simulink model "Batterymodel_HiL"  (Simulink 7.8)
settings: Solver=FixedStepDiscrete  SolverMode=SingleTasking  StartTime=0.0  StopTime=inf  FixedStep=T_s  RelTol=1e-3
PreLoadFcn:
  | //BatteryParameters;
  | Init_file_Bat
InitFcn:
  | Init_file_Bat;
values from neighbouring files (symbols this model uses):
  C_diff = 5000    [Init_file_Bat.m]
  CellNo = 12    [Init_file_Bat.m]
  ChargeCurrent = 5    [Init_file_Bat.m]
  ChargeSwitch = 1    [Init_file_Bat.m]
  DischargeCurrent = -5    [Init_file_Bat.m]
  n_cells = 12    [Init_file_Bat.m]
  poles_soc = polyfit(SoC_table, OCV_table,4)    [Init_file_Bat.m]
  Q_0 = 36000*ones(1,12)    [Init_file_Bat.m]
  R_ct = 3.2*10^-3    (= 0.0032)    [Init_file_Bat.m]
  R_diff = 4*10^-3    (= 0.004)    [Init_file_Bat.m]
  R_i = 2*10^-3    (= 0.002)    [Init_file_Bat.m]    (also in Kalman_para_int.m = single(0.05))
  SoCinitCells = SoC_init_cells    [Init_file_Bat.m]
  Tcells = T_cells    [Init_file_Bat.m]
  Ts = 10*10^-3    (= 0.01)    [Init_file_Bat.m]
undefined symbols (not defined in the file or in its folder): DiscIntNeverNeededParam, sigbuilder_block
(part 1 of 2)
settings Model: Creator=wezhang  LastModifiedBy=user  BufferReuse=off
settings OptimizationCC: BlockReduction=off  OptimizeBlockIOStorage=off  BufferReuse=off  ExpressionFolding=off  LocalBlockOutputs=off  InitFltsAndDblsToZero=on  SimCompilerOptimization=On
settings DebuggingCC: FcnCallInpInsideContextMsg=Use local settings
settings HardwareCC: ProdHWDeviceType=Generic->32-bit Embedded Processor
settings SFSimCC: SimParseCustomCode=off
settings RTWCC: SystemTargetFile=lcrt.tlc  GenCodeOnly=on  GenerateMakefile=off  TemplateMakefile=lcrt_default_tmf  GenerateReport=on  ProcessScript=lcrt_make_rtw_hook  LaunchReport=on  RTWCompilerOptimization=On
settings GRTTargetCC: UtilityFuncGeneration=Shared location  MatFileLogging=off  ExtModeMexFile=noextcomm

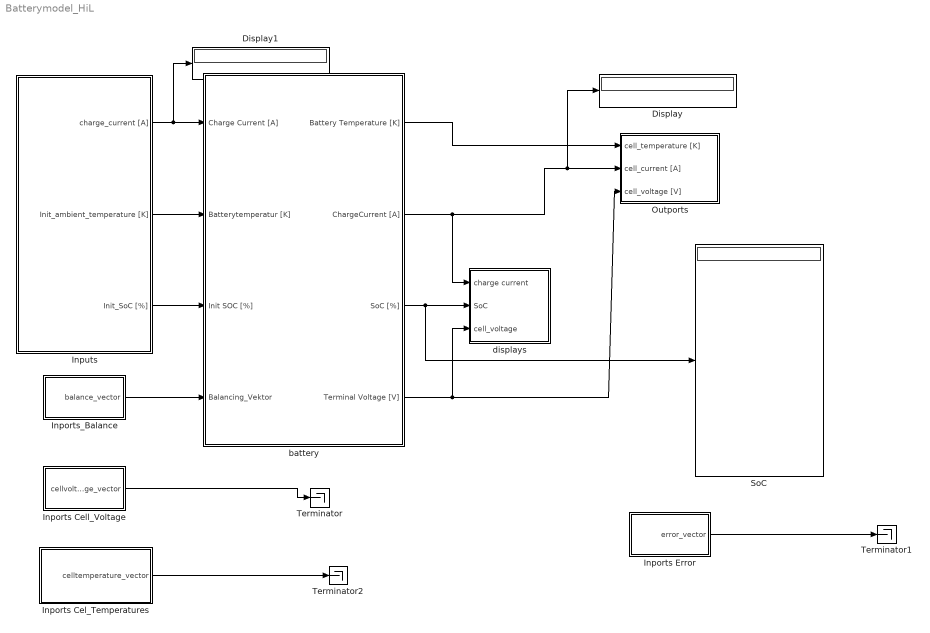
== system Batterymodel_HiL ==
  Display : Display
  Display1 : Display
  Inports Cel_Temperatures : Subsystem
  Inports Cell_Voltage : Subsystem
  Inports Error : Subsystem
  "Inports_Balance " : Subsystem
  Inputs : Subsystem
  Outports : Subsystem
  SoC : Display
  Terminator : Terminator
  Terminator1 : Terminator
  Terminator2 : Terminator
  battery : Subsystem
      settings: MinAlgLoopOccurrences=on
  displays : Subsystem
  wires:
  battery/1(Battery Temperature [K]) -> Outports/1(cell_temperature [K])
  battery/4(Terminal Voltage [V]) -> displays/3(cell_voltage), Outports/3(cell_voltage [V])
  battery/2(ChargeCurrent [A]) -> displays/1(charge current), Outports/2(cell_current [A]), Display/1
  Inputs/1(charge_current [A]) -> battery/1(Charge Current [A]), Display1/1
  Inputs/2(Init_ambient_temperature [K]) -> battery/2(Batterytemperatur [K])
  Inputs/3(Init_SoC [%]) -> battery/3(Init SOC [%])
  battery/3(SoC [%]) -> displays/2(SoC), SoC/1
  Inports Cell_Voltage/1(cellvoltage_vector) -> Terminator/1
  "Inports_Balance "/1(balance_vector) -> battery/4(Balancing_Vektor)
  Inports Error/1(error_vector) -> Terminator1/1
  Inports Cel_Temperatures/1(celltemperature_vector) -> Terminator2/1

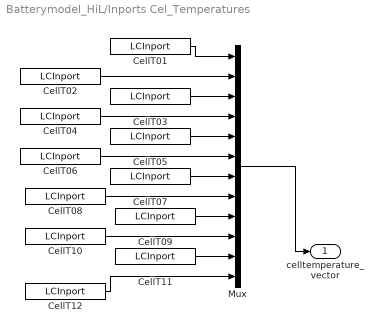
== system Batterymodel_HiL/Inports Cel_Temperatures ==
  CellT01 : S-Function  FunctionName=LCInport  Parameters=ModelName, InportID, b_useConstant, constValue  EnableBusSupport=off  mask(LABCAR Inport){ModelName='Batterymodel_HiL', InportID=0, b_useConstant=0, constValue=0}
      mask prompts: b_useConstant "Use Constant Value if Online"; constValue "Constant Value"
      mask help: This block gets an input to a Simulink model from another module of a LABCAR project
      settings: CopyFcn=set_param( gcb, 'UserData', '####');  OpenFcn=run LCInportGui
      mask Help:
      | Put this block onto any  hierarchy of the model and connect it to the model.
      | Rename it to any suitable name.
      | Then the corresponding signal is available in the Connection Manager for the wiring to any other module..
  CellT02 : S-Function  FunctionName=LCInport  Parameters=ModelName, InportID, b_useConstant, constValue  EnableBusSupport=off  mask(LABCAR Inport){ModelName='Batterymodel_HiL', InportID=1, b_useConstant=0, constValue=0}
      mask prompts: b_useConstant "Use Constant Value if Online"; constValue "Constant Value"
      mask help: This block gets an input to a Simulink model from another module of a LABCAR project
      settings: CopyFcn=set_param( gcb, 'UserData', '####');  OpenFcn=run LCInportGui
      mask Help:
      | Put this block onto any  hierarchy of the model and connect it to the model.
      | Rename it to any suitable name.
      | Then the corresponding signal is available in the Connection Manager for the wiring to any other module..
  CellT03 : S-Function  FunctionName=LCInport  Parameters=ModelName, InportID, b_useConstant, constValue  EnableBusSupport=off  mask(LABCAR Inport){ModelName='Batterymodel_HiL', InportID=2, b_useConstant=0, constValue=0}
      mask prompts: b_useConstant "Use Constant Value if Online"; constValue "Constant Value"
      mask help: This block gets an input to a Simulink model from another module of a LABCAR project
      settings: CopyFcn=set_param( gcb, 'UserData', '####');  OpenFcn=run LCInportGui
      mask Help:
      | Put this block onto any  hierarchy of the model and connect it to the model.
      | Rename it to any suitable name.
      | Then the corresponding signal is available in the Connection Manager for the wiring to any other module..
  CellT04 : S-Function  FunctionName=LCInport  Parameters=ModelName, InportID, b_useConstant, constValue  EnableBusSupport=off  mask(LABCAR Inport){ModelName='Batterymodel_HiL', InportID=3, b_useConstant=0, constValue=0}
      mask prompts: b_useConstant "Use Constant Value if Online"; constValue "Constant Value"
      mask help: This block gets an input to a Simulink model from another module of a LABCAR project
      settings: CopyFcn=set_param( gcb, 'UserData', '####');  OpenFcn=run LCInportGui
      mask Help:
      | Put this block onto any  hierarchy of the model and connect it to the model.
      | Rename it to any suitable name.
      | Then the corresponding signal is available in the Connection Manager for the wiring to any other module..
  CellT05 : S-Function  FunctionName=LCInport  Parameters=ModelName, InportID, b_useConstant, constValue  EnableBusSupport=off  mask(LABCAR Inport){ModelName='Batterymodel_HiL', InportID=4, b_useConstant=0, constValue=0}
      mask prompts: b_useConstant "Use Constant Value if Online"; constValue "Constant Value"
      mask help: This block gets an input to a Simulink model from another module of a LABCAR project
      settings: CopyFcn=set_param( gcb, 'UserData', '####');  OpenFcn=run LCInportGui
      mask Help:
      | Put this block onto any  hierarchy of the model and connect it to the model.
      | Rename it to any suitable name.
      | Then the corresponding signal is available in the Connection Manager for the wiring to any other module..
  CellT06 : S-Function  FunctionName=LCInport  Parameters=ModelName, InportID, b_useConstant, constValue  EnableBusSupport=off  mask(LABCAR Inport){ModelName='Batterymodel_HiL', InportID=5, b_useConstant=0, constValue=0}
      mask prompts: b_useConstant "Use Constant Value if Online"; constValue "Constant Value"
      mask help: This block gets an input to a Simulink model from another module of a LABCAR project
      settings: CopyFcn=set_param( gcb, 'UserData', '####');  OpenFcn=run LCInportGui
      mask Help:
      | Put this block onto any  hierarchy of the model and connect it to the model.
      | Rename it to any suitable name.
      | Then the corresponding signal is available in the Connection Manager for the wiring to any other module..
  CellT07 : S-Function  FunctionName=LCInport  Parameters=ModelName, InportID, b_useConstant, constValue  EnableBusSupport=off  mask(LABCAR Inport){ModelName='Batterymodel_HiL', InportID=6, b_useConstant=0, constValue=0}
      mask prompts: b_useConstant "Use Constant Value if Online"; constValue "Constant Value"
      mask help: This block gets an input to a Simulink model from another module of a LABCAR project
      settings: CopyFcn=set_param( gcb, 'UserData', '####');  OpenFcn=run LCInportGui
      mask Help:
      | Put this block onto any  hierarchy of the model and connect it to the model.
      | Rename it to any suitable name.
      | Then the corresponding signal is available in the Connection Manager for the wiring to any other module..
  CellT08 : S-Function  FunctionName=LCInport  Parameters=ModelName, InportID, b_useConstant, constValue  EnableBusSupport=off  mask(LABCAR Inport){ModelName='Batterymodel_HiL', InportID=7, b_useConstant=0, constValue=0}
      mask prompts: b_useConstant "Use Constant Value if Online"; constValue "Constant Value"
      mask help: This block gets an input to a Simulink model from another module of a LABCAR project
      settings: CopyFcn=set_param( gcb, 'UserData', '####');  OpenFcn=run LCInportGui
      mask Help:
      | Put this block onto any  hierarchy of the model and connect it to the model.
      | Rename it to any suitable name.
      | Then the corresponding signal is available in the Connection Manager for the wiring to any other module..
  CellT09 : S-Function  FunctionName=LCInport  Parameters=ModelName, InportID, b_useConstant, constValue  EnableBusSupport=off  mask(LABCAR Inport){ModelName='Batterymodel_HiL', InportID=8, b_useConstant=0, constValue=0}
      mask prompts: b_useConstant "Use Constant Value if Online"; constValue "Constant Value"
      mask help: This block gets an input to a Simulink model from another module of a LABCAR project
      settings: CopyFcn=set_param( gcb, 'UserData', '####');  OpenFcn=run LCInportGui
      mask Help:
      | Put this block onto any  hierarchy of the model and connect it to the model.
      | Rename it to any suitable name.
      | Then the corresponding signal is available in the Connection Manager for the wiring to any other module..
  CellT10 : S-Function  FunctionName=LCInport  Parameters=ModelName, InportID, b_useConstant, constValue  EnableBusSupport=off  mask(LABCAR Inport){ModelName='Batterymodel_HiL', InportID=9, b_useConstant=0, constValue=0}
      mask prompts: b_useConstant "Use Constant Value if Online"; constValue "Constant Value"
      mask help: This block gets an input to a Simulink model from another module of a LABCAR project
      settings: CopyFcn=set_param( gcb, 'UserData', '####');  OpenFcn=run LCInportGui
      mask Help:
      | Put this block onto any  hierarchy of the model and connect it to the model.
      | Rename it to any suitable name.
      | Then the corresponding signal is available in the Connection Manager for the wiring to any other module..
  CellT11 : S-Function  FunctionName=LCInport  Parameters=ModelName, InportID, b_useConstant, constValue  EnableBusSupport=off  mask(LABCAR Inport){ModelName='Batterymodel_HiL', InportID=10, b_useConstant=0, constValue=0}
      mask prompts: b_useConstant "Use Constant Value if Online"; constValue "Constant Value"
      mask help: This block gets an input to a Simulink model from another module of a LABCAR project
      settings: CopyFcn=set_param( gcb, 'UserData', '####');  OpenFcn=run LCInportGui
      mask Help:
      | Put this block onto any  hierarchy of the model and connect it to the model.
      | Rename it to any suitable name.
      | Then the corresponding signal is available in the Connection Manager for the wiring to any other module..
  CellT12 : S-Function  FunctionName=LCInport  Parameters=ModelName, InportID, b_useConstant, constValue  EnableBusSupport=off  mask(LABCAR Inport){ModelName='Batterymodel_HiL', InportID=11, b_useConstant=0, constValue=0}
      mask prompts: b_useConstant "Use Constant Value if Online"; constValue "Constant Value"
      mask help: This block gets an input to a Simulink model from another module of a LABCAR project
      settings: CopyFcn=set_param( gcb, 'UserData', '####');  OpenFcn=run LCInportGui
      mask Help:
      | Put this block onto any  hierarchy of the model and connect it to the model.
      | Rename it to any suitable name.
      | Then the corresponding signal is available in the Connection Manager for the wiring to any other module..
  Mux : Mux  Inputs=12
  celltemperature_vector : Outport
  wires:
  CellT01/1 -> Mux/1
  CellT02/1 -> Mux/2
  CellT03/1 -> Mux/3
  CellT04/1 -> Mux/4
  CellT05/1 -> Mux/5
  CellT06/1 -> Mux/6
  CellT08/1 -> Mux/8
  CellT10/1 -> Mux/10
  CellT12/1 -> Mux/12
  CellT11/1 -> Mux/11
  CellT09/1 -> Mux/9
  CellT07/1 -> Mux/7
  Mux/1 -> celltemperature_vector/1

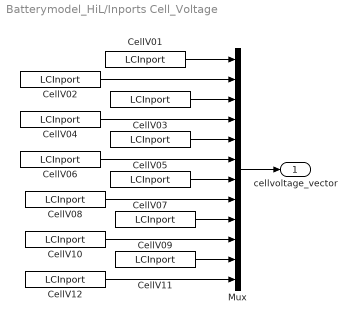
== system Batterymodel_HiL/Inports Cell_Voltage ==
  CellV01 : S-Function  FunctionName=LCInport  Parameters=ModelName, InportID, b_useConstant, constValue  EnableBusSupport=off  mask(LABCAR Inport){ModelName='Batterymodel_HiL', InportID=12, b_useConstant=0, constValue=0}
      mask prompts: b_useConstant "Use Constant Value if Online"; constValue "Constant Value"
      mask help: This block gets an input to a Simulink model from another module of a LABCAR project
      settings: CopyFcn=set_param( gcb, 'UserData', '####');  OpenFcn=run LCInportGui
      mask Help:
      | Put this block onto any  hierarchy of the model and connect it to the model.
      | Rename it to any suitable name.
      | Then the corresponding signal is available in the Connection Manager for the wiring to any other module..
  CellV02 : S-Function  FunctionName=LCInport  Parameters=ModelName, InportID, b_useConstant, constValue  EnableBusSupport=off  mask(LABCAR Inport){ModelName='Batterymodel_HiL', InportID=13, b_useConstant=0, constValue=0}
      mask prompts: b_useConstant "Use Constant Value if Online"; constValue "Constant Value"
      mask help: This block gets an input to a Simulink model from another module of a LABCAR project
      settings: CopyFcn=set_param( gcb, 'UserData', '####');  OpenFcn=run LCInportGui
      mask Help:
      | Put this block onto any  hierarchy of the model and connect it to the model.
      | Rename it to any suitable name.
      | Then the corresponding signal is available in the Connection Manager for the wiring to any other module..
  CellV03 : S-Function  FunctionName=LCInport  Parameters=ModelName, InportID, b_useConstant, constValue  EnableBusSupport=off  mask(LABCAR Inport){ModelName='Batterymodel_HiL', InportID=14, b_useConstant=0, constValue=0}
      mask prompts: b_useConstant "Use Constant Value if Online"; constValue "Constant Value"
      mask help: This block gets an input to a Simulink model from another module of a LABCAR project
      settings: CopyFcn=set_param( gcb, 'UserData', '####');  OpenFcn=run LCInportGui
      mask Help:
      | Put this block onto any  hierarchy of the model and connect it to the model.
      | Rename it to any suitable name.
      | Then the corresponding signal is available in the Connection Manager for the wiring to any other module..
  CellV04 : S-Function  FunctionName=LCInport  Parameters=ModelName, InportID, b_useConstant, constValue  EnableBusSupport=off  mask(LABCAR Inport){ModelName='Batterymodel_HiL', InportID=15, b_useConstant=0, constValue=0}
      mask prompts: b_useConstant "Use Constant Value if Online"; constValue "Constant Value"
      mask help: This block gets an input to a Simulink model from another module of a LABCAR project
      settings: CopyFcn=set_param( gcb, 'UserData', '####');  OpenFcn=run LCInportGui
      mask Help:
      | Put this block onto any  hierarchy of the model and connect it to the model.
      | Rename it to any suitable name.
      | Then the corresponding signal is available in the Connection Manager for the wiring to any other module..
  CellV05 : S-Function  FunctionName=LCInport  Parameters=ModelName, InportID, b_useConstant, constValue  EnableBusSupport=off  mask(LABCAR Inport){ModelName='Batterymodel_HiL', InportID=16, b_useConstant=0, constValue=0}
      mask prompts: b_useConstant "Use Constant Value if Online"; constValue "Constant Value"
      mask help: This block gets an input to a Simulink model from another module of a LABCAR project
      settings: CopyFcn=set_param( gcb, 'UserData', '####');  OpenFcn=run LCInportGui
      mask Help:
      | Put this block onto any  hierarchy of the model and connect it to the model.
      | Rename it to any suitable name.
      | Then the corresponding signal is available in the Connection Manager for the wiring to any other module..
  CellV06 : S-Function  FunctionName=LCInport  Parameters=ModelName, InportID, b_useConstant, constValue  EnableBusSupport=off  mask(LABCAR Inport){ModelName='Batterymodel_HiL', InportID=17, b_useConstant=0, constValue=0}
      mask prompts: b_useConstant "Use Constant Value if Online"; constValue "Constant Value"
      mask help: This block gets an input to a Simulink model from another module of a LABCAR project
      settings: CopyFcn=set_param( gcb, 'UserData', '####');  OpenFcn=run LCInportGui
      mask Help:
      | Put this block onto any  hierarchy of the model and connect it to the model.
      | Rename it to any suitable name.
      | Then the corresponding signal is available in the Connection Manager for the wiring to any other module..
  CellV07 : S-Function  FunctionName=LCInport  Parameters=ModelName, InportID, b_useConstant, constValue  EnableBusSupport=off  mask(LABCAR Inport){ModelName='Batterymodel_HiL', InportID=18, b_useConstant=0, constValue=0}
      mask prompts: b_useConstant "Use Constant Value if Online"; constValue "Constant Value"
      mask help: This block gets an input to a Simulink model from another module of a LABCAR project
      settings: CopyFcn=set_param( gcb, 'UserData', '####');  OpenFcn=run LCInportGui
      mask Help:
      | Put this block onto any  hierarchy of the model and connect it to the model.
      | Rename it to any suitable name.
      | Then the corresponding signal is available in the Connection Manager for the wiring to any other module..
  CellV08 : S-Function  FunctionName=LCInport  Parameters=ModelName, InportID, b_useConstant, constValue  EnableBusSupport=off  mask(LABCAR Inport){ModelName='Batterymodel_HiL', InportID=19, b_useConstant=0, constValue=0}
      mask prompts: b_useConstant "Use Constant Value if Online"; constValue "Constant Value"
      mask help: This block gets an input to a Simulink model from another module of a LABCAR project
      settings: CopyFcn=set_param( gcb, 'UserData', '####');  OpenFcn=run LCInportGui
      mask Help:
      | Put this block onto any  hierarchy of the model and connect it to the model.
      | Rename it to any suitable name.
      | Then the corresponding signal is available in the Connection Manager for the wiring to any other module..
  CellV09 : S-Function  FunctionName=LCInport  Parameters=ModelName, InportID, b_useConstant, constValue  EnableBusSupport=off  mask(LABCAR Inport){ModelName='Batterymodel_HiL', InportID=20, b_useConstant=0, constValue=0}
      mask prompts: b_useConstant "Use Constant Value if Online"; constValue "Constant Value"
      mask help: This block gets an input to a Simulink model from another module of a LABCAR project
      settings: CopyFcn=set_param( gcb, 'UserData', '####');  OpenFcn=run LCInportGui
      mask Help:
      | Put this block onto any  hierarchy of the model and connect it to the model.
      | Rename it to any suitable name.
      | Then the corresponding signal is available in the Connection Manager for the wiring to any other module..
  CellV10 : S-Function  FunctionName=LCInport  Parameters=ModelName, InportID, b_useConstant, constValue  EnableBusSupport=off  mask(LABCAR Inport){ModelName='Batterymodel_HiL', InportID=21, b_useConstant=0, constValue=0}
      mask prompts: b_useConstant "Use Constant Value if Online"; constValue "Constant Value"
      mask help: This block gets an input to a Simulink model from another module of a LABCAR project
      settings: CopyFcn=set_param( gcb, 'UserData', '####');  OpenFcn=run LCInportGui
      mask Help:
      | Put this block onto any  hierarchy of the model and connect it to the model.
      | Rename it to any suitable name.
      | Then the corresponding signal is available in the Connection Manager for the wiring to any other module..
  CellV11 : S-Function  FunctionName=LCInport  Parameters=ModelName, InportID, b_useConstant, constValue  EnableBusSupport=off  mask(LABCAR Inport){ModelName='Batterymodel_HiL', InportID=22, b_useConstant=0, constValue=0}
      mask prompts: b_useConstant "Use Constant Value if Online"; constValue "Constant Value"
      mask help: This block gets an input to a Simulink model from another module of a LABCAR project
      settings: CopyFcn=set_param( gcb, 'UserData', '####');  OpenFcn=run LCInportGui
      mask Help:
      | Put this block onto any  hierarchy of the model and connect it to the model.
      | Rename it to any suitable name.
      | Then the corresponding signal is available in the Connection Manager for the wiring to any other module..
  CellV12 : S-Function  FunctionName=LCInport  Parameters=ModelName, InportID, b_useConstant, constValue  EnableBusSupport=off  mask(LABCAR Inport){ModelName='Batterymodel_HiL', InportID=23, b_useConstant=0, constValue=0}
      mask prompts: b_useConstant "Use Constant Value if Online"; constValue "Constant Value"
      mask help: This block gets an input to a Simulink model from another module of a LABCAR project
      settings: CopyFcn=set_param( gcb, 'UserData', '####');  OpenFcn=run LCInportGui
      mask Help:
      | Put this block onto any  hierarchy of the model and connect it to the model.
      | Rename it to any suitable name.
      | Then the corresponding signal is available in the Connection Manager for the wiring to any other module..
  Mux : Mux  Inputs=12
  cellvoltage_vector : Outport
  wires:
  CellV01/1 -> Mux/1
  CellV02/1 -> Mux/2
  CellV03/1 -> Mux/3
  CellV04/1 -> Mux/4
  CellV05/1 -> Mux/5
  CellV06/1 -> Mux/6
  CellV08/1 -> Mux/8
  CellV10/1 -> Mux/10
  CellV12/1 -> Mux/12
  CellV11/1 -> Mux/11
  CellV09/1 -> Mux/9
  CellV07/1 -> Mux/7
  Mux/1 -> cellvoltage_vector/1

== system Batterymodel_HiL/Inports Error ==
  Error_CellNo : S-Function  FunctionName=LCInport  Parameters=ModelName, InportID, b_useConstant, constValue  EnableBusSupport=off  mask(LABCAR Inport){ModelName='Batterymodel_HiL', InportID=24, b_useConstant=0, constValue=0}
      mask prompts: b_useConstant "Use Constant Value if Online"; constValue "Constant Value"
      mask help: This block gets an input to a Simulink model from another module of a LABCAR project
      settings: CopyFcn=set_param( gcb, 'UserData', '####');  OpenFcn=run LCInportGui
      mask Help:
      | Put this block onto any  hierarchy of the model and connect it to the model.
      | Rename it to any suitable name.
      | Then the corresponding signal is available in the Connection Manager for the wiring to any other module..
  Error_Event : S-Function  FunctionName=LCInport  Parameters=ModelName, InportID, b_useConstant, constValue  EnableBusSupport=off  mask(LABCAR Inport){ModelName='Batterymodel_HiL', InportID=25, b_useConstant=0, constValue=0}
      mask prompts: b_useConstant "Use Constant Value if Online"; constValue "Constant Value"
      mask help: This block gets an input to a Simulink model from another module of a LABCAR project
      settings: CopyFcn=set_param( gcb, 'UserData', '####');  OpenFcn=run LCInportGui
      mask Help:
      | Put this block onto any  hierarchy of the model and connect it to the model.
      | Rename it to any suitable name.
      | Then the corresponding signal is available in the Connection Manager for the wiring to any other module..
  Error_Indication : S-Function  FunctionName=LCInport  Parameters=ModelName, InportID, b_useConstant, constValue  EnableBusSupport=off  mask(LABCAR Inport){ModelName='Batterymodel_HiL', InportID=26, b_useConstant=0, constValue=0}
      mask prompts: b_useConstant "Use Constant Value if Online"; constValue "Constant Value"
      mask help: This block gets an input to a Simulink model from another module of a LABCAR project
      settings: CopyFcn=set_param( gcb, 'UserData', '####');  OpenFcn=run LCInportGui
      mask Help:
      | Put this block onto any  hierarchy of the model and connect it to the model.
      | Rename it to any suitable name.
      | Then the corresponding signal is available in the Connection Manager for the wiring to any other module..
  Mux : Mux  Inputs=3
  error_vector : Outport
  wires:
  Error_Indication/1 -> Mux/1
  Error_Event/1 -> Mux/2
  Error_CellNo/1 -> Mux/3
  Mux/1 -> error_vector/1

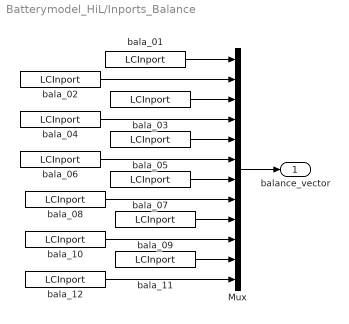
== system Batterymodel_HiL/Inports_Balance  ==
  Mux : Mux  Inputs=12
  bala_01 : S-Function  FunctionName=LCInport  Parameters=ModelName, InportID, b_useConstant, constValue  EnableBusSupport=off  mask(LABCAR Inport){ModelName='Batterymodel_HiL', InportID=27, b_useConstant=0, constValue=0}
      mask prompts: b_useConstant "Use Constant Value if Online"; constValue "Constant Value"
      mask help: This block gets an input to a Simulink model from another module of a LABCAR project
      settings: CopyFcn=set_param( gcb, 'UserData', '####');  OpenFcn=run LCInportGui
      mask Help:
      | Put this block onto any  hierarchy of the model and connect it to the model.
      | Rename it to any suitable name.
      | Then the corresponding signal is available in the Connection Manager for the wiring to any other module..
  bala_02 : S-Function  FunctionName=LCInport  Parameters=ModelName, InportID, b_useConstant, constValue  EnableBusSupport=off  mask(LABCAR Inport){ModelName='Batterymodel_HiL', InportID=28, b_useConstant=0, constValue=0}
      mask prompts: b_useConstant "Use Constant Value if Online"; constValue "Constant Value"
      mask help: This block gets an input to a Simulink model from another module of a LABCAR project
      settings: CopyFcn=set_param( gcb, 'UserData', '####');  OpenFcn=run LCInportGui
      mask Help:
      | Put this block onto any  hierarchy of the model and connect it to the model.
      | Rename it to any suitable name.
      | Then the corresponding signal is available in the Connection Manager for the wiring to any other module..
  bala_03 : S-Function  FunctionName=LCInport  Parameters=ModelName, InportID, b_useConstant, constValue  EnableBusSupport=off  mask(LABCAR Inport){ModelName='Batterymodel_HiL', InportID=29, b_useConstant=0, constValue=0}
      mask prompts: b_useConstant "Use Constant Value if Online"; constValue "Constant Value"
      mask help: This block gets an input to a Simulink model from another module of a LABCAR project
      settings: CopyFcn=set_param( gcb, 'UserData', '####');  OpenFcn=run LCInportGui
      mask Help:
      | Put this block onto any  hierarchy of the model and connect it to the model.
      | Rename it to any suitable name.
      | Then the corresponding signal is available in the Connection Manager for the wiring to any other module..
  bala_04 : S-Function  FunctionName=LCInport  Parameters=ModelName, InportID, b_useConstant, constValue  EnableBusSupport=off  mask(LABCAR Inport){ModelName='Batterymodel_HiL', InportID=30, b_useConstant=0, constValue=0}
      mask prompts: b_useConstant "Use Constant Value if Online"; constValue "Constant Value"
      mask help: This block gets an input to a Simulink model from another module of a LABCAR project
      settings: CopyFcn=set_param( gcb, 'UserData', '####');  OpenFcn=run LCInportGui
      mask Help:
      | Put this block onto any  hierarchy of the model and connect it to the model.
      | Rename it to any suitable name.
      | Then the corresponding signal is available in the Connection Manager for the wiring to any other module..
  bala_05 : S-Function  FunctionName=LCInport  Parameters=ModelName, InportID, b_useConstant, constValue  EnableBusSupport=off  mask(LABCAR Inport){ModelName='Batterymodel_HiL', InportID=31, b_useConstant=0, constValue=0}
      mask prompts: b_useConstant "Use Constant Value if Online"; constValue "Constant Value"
      mask help: This block gets an input to a Simulink model from another module of a LABCAR project
      settings: CopyFcn=set_param( gcb, 'UserData', '####');  OpenFcn=run LCInportGui
      mask Help:
      | Put this block onto any  hierarchy of the model and connect it to the model.
      | Rename it to any suitable name.
      | Then the corresponding signal is available in the Connection Manager for the wiring to any other module..
  bala_06 : S-Function  FunctionName=LCInport  Parameters=ModelName, InportID, b_useConstant, constValue  EnableBusSupport=off  mask(LABCAR Inport){ModelName='Batterymodel_HiL', InportID=32, b_useConstant=0, constValue=0}
      mask prompts: b_useConstant "Use Constant Value if Online"; constValue "Constant Value"
      mask help: This block gets an input to a Simulink model from another module of a LABCAR project
      settings: CopyFcn=set_param( gcb, 'UserData', '####');  OpenFcn=run LCInportGui
      mask Help:
      | Put this block onto any  hierarchy of the model and connect it to the model.
      | Rename it to any suitable name.
      | Then the corresponding signal is available in the Connection Manager for the wiring to any other module..
  bala_07 : S-Function  FunctionName=LCInport  Parameters=ModelName, InportID, b_useConstant, constValue  EnableBusSupport=off  mask(LABCAR Inport){ModelName='Batterymodel_HiL', InportID=33, b_useConstant=0, constValue=0}
      mask prompts: b_useConstant "Use Constant Value if Online"; constValue "Constant Value"
      mask help: This block gets an input to a Simulink model from another module of a LABCAR project
      settings: CopyFcn=set_param( gcb, 'UserData', '####');  OpenFcn=run LCInportGui
      mask Help:
      | Put this block onto any  hierarchy of the model and connect it to the model.
      | Rename it to any suitable name.
      | Then the corresponding signal is available in the Connection Manager for the wiring to any other module..
  bala_08 : S-Function  FunctionName=LCInport  Parameters=ModelName, InportID, b_useConstant, constValue  EnableBusSupport=off  mask(LABCAR Inport){ModelName='Batterymodel_HiL', InportID=34, b_useConstant=0, constValue=0}
      mask prompts: b_useConstant "Use Constant Value if Online"; constValue "Constant Value"
      mask help: This block gets an input to a Simulink model from another module of a LABCAR project
      settings: CopyFcn=set_param( gcb, 'UserData', '####');  OpenFcn=run LCInportGui
      mask Help:
      | Put this block onto any  hierarchy of the model and connect it to the model.
      | Rename it to any suitable name.
      | Then the corresponding signal is available in the Connection Manager for the wiring to any other module..
  bala_09 : S-Function  FunctionName=LCInport  Parameters=ModelName, InportID, b_useConstant, constValue  EnableBusSupport=off  mask(LABCAR Inport){ModelName='Batterymodel_HiL', InportID=35, b_useConstant=0, constValue=0}
      mask prompts: b_useConstant "Use Constant Value if Online"; constValue "Constant Value"
      mask help: This block gets an input to a Simulink model from another module of a LABCAR project
      settings: CopyFcn=set_param( gcb, 'UserData', '####');  OpenFcn=run LCInportGui
      mask Help:
      | Put this block onto any  hierarchy of the model and connect it to the model.
      | Rename it to any suitable name.
      | Then the corresponding signal is available in the Connection Manager for the wiring to any other module..
  bala_10 : S-Function  FunctionName=LCInport  Parameters=ModelName, InportID, b_useConstant, constValue  EnableBusSupport=off  mask(LABCAR Inport){ModelName='Batterymodel_HiL', InportID=36, b_useConstant=0, constValue=0}
      mask prompts: b_useConstant "Use Constant Value if Online"; constValue "Constant Value"
      mask help: This block gets an input to a Simulink model from another module of a LABCAR project
      settings: CopyFcn=set_param( gcb, 'UserData', '####');  OpenFcn=run LCInportGui
      mask Help:
      | Put this block onto any  hierarchy of the model and connect it to the model.
      | Rename it to any suitable name.
      | Then the corresponding signal is available in the Connection Manager for the wiring to any other module..
  bala_11 : S-Function  FunctionName=LCInport  Parameters=ModelName, InportID, b_useConstant, constValue  EnableBusSupport=off  mask(LABCAR Inport){ModelName='Batterymodel_HiL', InportID=37, b_useConstant=0, constValue=0}
      mask prompts: b_useConstant "Use Constant Value if Online"; constValue "Constant Value"
      mask help: This block gets an input to a Simulink model from another module of a LABCAR project
      settings: CopyFcn=set_param( gcb, 'UserData', '####');  OpenFcn=run LCInportGui
      mask Help:
      | Put this block onto any  hierarchy of the model and connect it to the model.
      | Rename it to any suitable name.
      | Then the corresponding signal is available in the Connection Manager for the wiring to any other module..
  bala_12 : S-Function  FunctionName=LCInport  Parameters=ModelName, InportID, b_useConstant, constValue  EnableBusSupport=off  mask(LABCAR Inport){ModelName='Batterymodel_HiL', InportID=38, b_useConstant=0, constValue=0}
      mask prompts: b_useConstant "Use Constant Value if Online"; constValue "Constant Value"
      mask help: This block gets an input to a Simulink model from another module of a LABCAR project
      settings: CopyFcn=set_param( gcb, 'UserData', '####');  OpenFcn=run LCInportGui
      mask Help:
      | Put this block onto any  hierarchy of the model and connect it to the model.
      | Rename it to any suitable name.
      | Then the corresponding signal is available in the Connection Manager for the wiring to any other module..
  balance_vector : Outport
  wires:
  bala_01/1 -> Mux/1
  bala_02/1 -> Mux/2
  bala_03/1 -> Mux/3
  bala_04/1 -> Mux/4
  bala_05/1 -> Mux/5
  bala_06/1 -> Mux/6
  bala_08/1 -> Mux/8
  bala_10/1 -> Mux/10
  bala_12/1 -> Mux/12
  bala_11/1 -> Mux/11
  bala_09/1 -> Mux/9
  bala_07/1 -> Mux/7
  Mux/1 -> balance_vector/1

== system Batterymodel_HiL/Inputs ==
  Betriebsmodus : Subsystem
  Charge Profile : Subsystem
  Init Ambient Temperature [K] : Constant  Value=Tcells
  Init SoC [%] : Constant  Value=SoCinitCells
  charge_current [A] : Outport
  Init_ambient_temperature [K] : Outport  Port=2
  Init_SoC [%] : Outport  Port=3
  wires:
  Charge Profile/1(Current [A]) -> charge_current [A]/1
  Init Ambient Temperature [K]/1 -> Init_ambient_temperature [K]/1
  Init SoC [%]/1 -> Init_SoC [%]/1

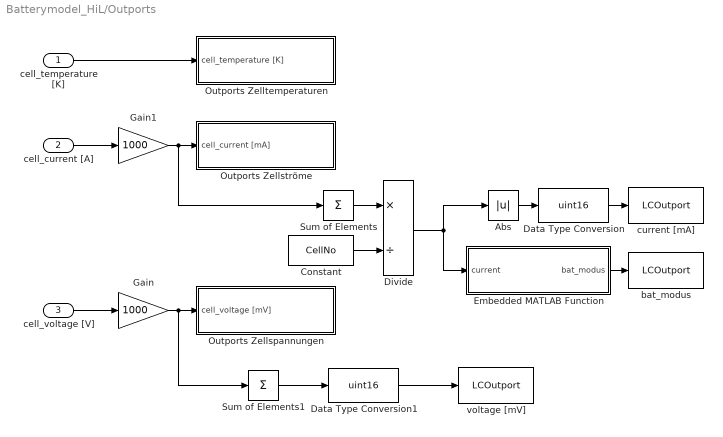
== system Batterymodel_HiL/Outports ==
  cell_temperature [K] : Inport
  cell_current [A] : Inport  Port=2
  cell_voltage [V] : Inport  Port=3
  Abs : Abs
  Constant : Constant  Value=CellNo
  Data Type Conversion : DataTypeConversion  OutDataTypeStr=uint16
  Data Type Conversion1 : DataTypeConversion  OutDataTypeStr=uint16
  Divide : Product  Inputs=*/
  Embedded MATLAB Function : MATLAB Function  TreatAsAtomicUnit=on
  Gain : Gain  Gain=1000
  Gain1 : Gain  Gain=1000
  Outports Zellspannungen : Subsystem
  Outports Zellströme : Subsystem
  Outports Zelltemperaturen : Subsystem
  Sum of Elements : Sum  Inputs=+
  Sum of Elements1 : Sum  Inputs=+
  bat_modus : S-Function  FunctionName=LCOutport  Parameters=ModelName, OutportID  EnableBusSupport=off  mask(LABCAR Outport){ModelName='Batterymodel_HiL', OutportID=37}
      mask help: This block defines an output of a Simulink model to another module of a LABCAR project
      settings: CopyFcn=set_param( gcb, 'UserData', '####');  OpenFcn=LCOpenFcnCallback
      mask Help:
      | Put this block onto any  hierarchy of the model and connect it to the model.
      | Rename it to any suitable name.
      | Then the corresponding signal is available in the Connection Manager for the wiring to any other module..
  current [mA] : S-Function  FunctionName=LCOutport  Parameters=ModelName, OutportID  EnableBusSupport=off  mask(LABCAR Outport){ModelName='Batterymodel_HiL', OutportID=38}
      mask help: This block defines an output of a Simulink model to another module of a LABCAR project
      settings: CopyFcn=set_param( gcb, 'UserData', '####');  OpenFcn=LCOpenFcnCallback
      mask Help:
      | Put this block onto any  hierarchy of the model and connect it to the model.
      | Rename it to any suitable name.
      | Then the corresponding signal is available in the Connection Manager for the wiring to any other module..
  voltage [mV] : S-Function  FunctionName=LCOutport  Parameters=ModelName, OutportID  EnableBusSupport=off  mask(LABCAR Outport){ModelName='Batterymodel_HiL', OutportID=39}
      mask help: This block defines an output of a Simulink model to another module of a LABCAR project
      settings: CopyFcn=set_param( gcb, 'UserData', '####');  OpenFcn=LCOpenFcnCallback
      mask Help:
      | Put this block onto any  hierarchy of the model and connect it to the model.
      | Rename it to any suitable name.
      | Then the corresponding signal is available in the Connection Manager for the wiring to any other module..
  wires:
  Gain/1 -> Outports Zellspannungen/1(cell_voltage [mV]), Sum of Elements1/1
  cell_voltage [V]/1 -> Gain/1
  cell_temperature [K]/1 -> Outports Zelltemperaturen/1(cell_temperature [K])
  cell_current [A]/1 -> Gain1/1
  Sum of Elements/1 -> Divide/1
  Constant/1 -> Divide/2
  Gain1/1 -> Outports Zellströme/1(cell_current [mA]), Sum of Elements/1
  Sum of Elements1/1 -> Data Type Conversion1/1
  Abs/1 -> Data Type Conversion/1
  Divide/1 -> Embedded MATLAB Function/1(current), Abs/1
  Embedded MATLAB Function/1(bat_modus) -> bat_modus/1
  Data Type Conversion/1 -> current [mA]/1
  Data Type Conversion1/1 -> voltage [mV]/1

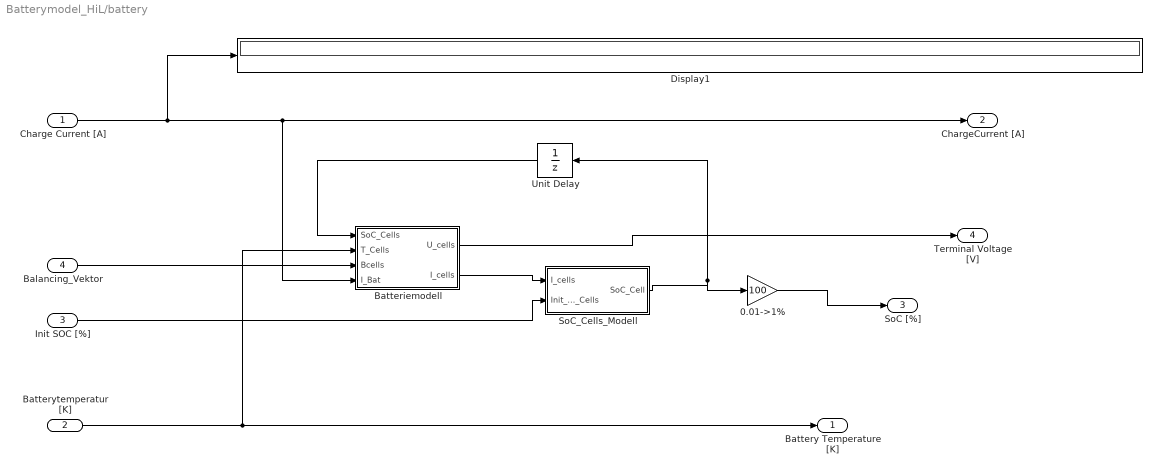
== system Batterymodel_HiL/battery ==
  Charge Current [A] : Inport
  Batterytemperatur [K] : Inport  Port=2
  Init SOC [%] : Inport  Port=3
  Balancing_Vektor : Inport  Port=4
  0.01->1% : Gain  Gain=100
  Batteriemodell : Subsystem
  Display1 : Display
  SoC_Cells_Modell : Subsystem
  Unit Delay : UnitDelay  SampleTime=-1
  Battery Temperature [K] : Outport
  ChargeCurrent [A] : Outport  Port=2
  SoC [%] : Outport  Port=3
  Terminal Voltage [V] : Outport  Port=4
  wires:
  Charge Current [A]/1 -> Batteriemodell/4(I_Bat), ChargeCurrent [A]/1, Display1/1
  Batteriemodell/2(I_cells) -> SoC_Cells_Modell/1(I_cells)
  SoC_Cells_Modell/1(SoC_Cell) -> Unit Delay/1, 0.01->1%/1
  Batteriemodell/1(U_cells) -> Terminal Voltage [V]/1
  Batterytemperatur [K]/1 -> Batteriemodell/2(T_Cells), Battery Temperature [K]/1
  Init SOC [%]/1 -> SoC_Cells_Modell/2(Init_SoC_Cells)
  Balancing_Vektor/1 -> Batteriemodell/3(Bcells)
  Unit Delay/1 -> Batteriemodell/1(SoC_Cells)
  0.01->1%/1 -> SoC [%]/1

== system Batterymodel_HiL/displays ==
  charge current : Inport
  SoC : Inport  Port=2
  cell_voltage : Inport  Port=3
  Batteirespannung : Subsystem
  Batteriestrom : Subsystem
  Vergleich SoC : Subsystem
  wires:
  cell_voltage/1 -> Batteirespannung/1(cell_voltage [V])
  charge current/1 -> Batteriestrom/1(charge current [A])
  SoC/1 -> Vergleich SoC/1(SoC Modell [%])

== system Batterymodel_HiL/Inputs/Betriebsmodus ==
  Mod_CAN_RS232 : Constant  Value=0
  Mod_CAN_RS232_Com : S-Function  FunctionName=LCOutport  Parameters=ModelName, OutportID  EnableBusSupport=off  mask(LABCAR Outport){ModelName='Batterymodel_HiL', OutportID=0}
      mask help: This block defines an output of a Simulink model to another module of a LABCAR project
      settings: CopyFcn=set_param( gcb, 'UserData', '####');  OpenFcn=LCOpenFcnCallback
      mask Help:
      | Put this block onto any  hierarchy of the model and connect it to the model.
      | Rename it to any suitable name.
      | Then the corresponding signal is available in the Connection Manager for the wiring to any other module..
  wires:
  Mod_CAN_RS232/1 -> Mod_CAN_RS232_Com/1

== system Batterymodel_HiL/Inputs/Charge Profile ==
  ChargeCurrent[A] : Constant  Value=ChargeCurrent
  ChargeCurrent[A]1 : Constant  Value=DischargeCurrent
  ChargeSwitch : Constant  Value=ChargeSwitch
  Constant1 : Constant  Value=ones(CellNo,1)
  Multiport Switch : MultiPortSwitch  zeroidx=off  InputSameDT=on
  Product : Product  RndMeth=Zero
  virtuel drive cycle : Subsystem  Tag=STV Subsys  LoadFcn=sigbuilder_block('load');  StartFcn=sigbuilder_block('start');  StopFcn=sigbuilder_block('stop');  ClipboardFcn=sigbuilder_block('clipboard');  mask(Sigbuilder block){}
      mask help: Sigbuilder GUI
      mask init:
      | if ~strcmp(get_param(bdroot(gcbh),'SimulationStatus'),'stopped') tuvar = sigbuilder_block('maskInit'); end
      settings: CopyFcn=sigbuilder_block('copy');  DeleteFcn=sigbuilder_block('delete');  ModelCloseFcn=sigbuilder_block('modelClose');  PreSaveFcn=sigbuilder_block('preSave');  NameChangeFcn=sigbuilder_block('namechange');  OpenFcn=sigbuilder_block('open',[72.75 6 756 453 ]);  CloseFcn=sigbuilder_block('close');
      mask Display: plot(0,0,100,100,[10,10,40,40,10],[80,20,20,80,80],[40,10],[50,50], [40,27,10],[65,72,56],[40,25,25,10],[28,28,43,43]);
  Current [A] : Outport
  wires:
  Multiport Switch/1 -> Product/1  "ChargeCurrent[A]"
  ChargeSwitch/1 -> Multiport Switch/1
  ChargeCurrent[A]1/1 -> Multiport Switch/2
  ChargeCurrent[A]/1 -> Multiport Switch/3
  Constant1/1 -> Product/2
  Product/1 -> Current [A]/1  "ChargeCurrent[A]"
  virtuel drive cycle/1(Signal 1) -> Multiport Switch/4

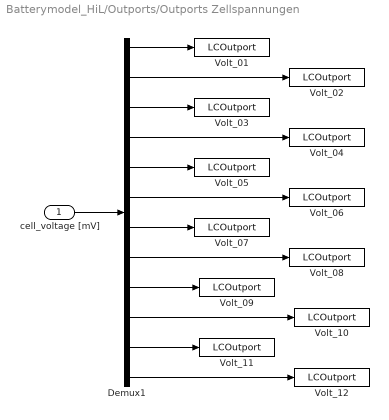
== system Batterymodel_HiL/Outports/Outports Zellspannungen ==
  cell_voltage [mV] : Inport
  Demux1 : Demux  Outputs=12
  Volt_01 : S-Function  FunctionName=LCOutport  Parameters=ModelName, OutportID  EnableBusSupport=off  mask(LABCAR Outport){ModelName='Batterymodel_HiL', OutportID=1}
      mask help: This block defines an output of a Simulink model to another module of a LABCAR project
      settings: CopyFcn=set_param( gcb, 'UserData', '####');  OpenFcn=LCOpenFcnCallback
      mask Help:
      | Put this block onto any  hierarchy of the model and connect it to the model.
      | Rename it to any suitable name.
      | Then the corresponding signal is available in the Connection Manager for the wiring to any other module..
  Volt_02 : S-Function  FunctionName=LCOutport  Parameters=ModelName, OutportID  EnableBusSupport=off  mask(LABCAR Outport){ModelName='Batterymodel_HiL', OutportID=2}
      mask help: This block defines an output of a Simulink model to another module of a LABCAR project
      settings: CopyFcn=set_param( gcb, 'UserData', '####');  OpenFcn=LCOpenFcnCallback
      mask Help:
      | Put this block onto any  hierarchy of the model and connect it to the model.
      | Rename it to any suitable name.
      | Then the corresponding signal is available in the Connection Manager for the wiring to any other module..
  Volt_03 : S-Function  FunctionName=LCOutport  Parameters=ModelName, OutportID  EnableBusSupport=off  mask(LABCAR Outport){ModelName='Batterymodel_HiL', OutportID=3}
      mask help: This block defines an output of a Simulink model to another module of a LABCAR project
      settings: CopyFcn=set_param( gcb, 'UserData', '####');  OpenFcn=LCOpenFcnCallback
      mask Help:
      | Put this block onto any  hierarchy of the model and connect it to the model.
      | Rename it to any suitable name.
      | Then the corresponding signal is available in the Connection Manager for the wiring to any other module..
  Volt_04 : S-Function  FunctionName=LCOutport  Parameters=ModelName, OutportID  EnableBusSupport=off  mask(LABCAR Outport){ModelName='Batterymodel_HiL', OutportID=4}
      mask help: This block defines an output of a Simulink model to another module of a LABCAR project
      settings: CopyFcn=set_param( gcb, 'UserData', '####');  OpenFcn=LCOpenFcnCallback
      mask Help:
      | Put this block onto any  hierarchy of the model and connect it to the model.
      | Rename it to any suitable name.
      | Then the corresponding signal is available in the Connection Manager for the wiring to any other module..
  Volt_05 : S-Function  FunctionName=LCOutport  Parameters=ModelName, OutportID  EnableBusSupport=off  mask(LABCAR Outport){ModelName='Batterymodel_HiL', OutportID=5}
      mask help: This block defines an output of a Simulink model to another module of a LABCAR project
      settings: CopyFcn=set_param( gcb, 'UserData', '####');  OpenFcn=LCOpenFcnCallback
      mask Help:
      | Put this block onto any  hierarchy of the model and connect it to the model.
      | Rename it to any suitable name.
      | Then the corresponding signal is available in the Connection Manager for the wiring to any other module..
  Volt_06 : S-Function  FunctionName=LCOutport  Parameters=ModelName, OutportID  EnableBusSupport=off  mask(LABCAR Outport){ModelName='Batterymodel_HiL', OutportID=6}
      mask help: This block defines an output of a Simulink model to another module of a LABCAR project
      settings: CopyFcn=set_param( gcb, 'UserData', '####');  OpenFcn=LCOpenFcnCallback
      mask Help:
      | Put this block onto any  hierarchy of the model and connect it to the model.
      | Rename it to any suitable name.
      | Then the corresponding signal is available in the Connection Manager for the wiring to any other module..
  Volt_07 : S-Function  FunctionName=LCOutport  Parameters=ModelName, OutportID  EnableBusSupport=off  mask(LABCAR Outport){ModelName='Batterymodel_HiL', OutportID=7}
      mask help: This block defines an output of a Simulink model to another module of a LABCAR project
      settings: CopyFcn=set_param( gcb, 'UserData', '####');  OpenFcn=LCOpenFcnCallback
      mask Help:
      | Put this block onto any  hierarchy of the model and connect it to the model.
      | Rename it to any suitable name.
      | Then the corresponding signal is available in the Connection Manager for the wiring to any other module..
  Volt_08 : S-Function  FunctionName=LCOutport  Parameters=ModelName, OutportID  EnableBusSupport=off  mask(LABCAR Outport){ModelName='Batterymodel_HiL', OutportID=8}
      mask help: This block defines an output of a Simulink model to another module of a LABCAR project
      settings: CopyFcn=set_param( gcb, 'UserData', '####');  OpenFcn=LCOpenFcnCallback
      mask Help:
      | Put this block onto any  hierarchy of the model and connect it to the model.
      | Rename it to any suitable name.
      | Then the corresponding signal is available in the Connection Manager for the wiring to any other module..
  Volt_09 : S-Function  FunctionName=LCOutport  Parameters=ModelName, OutportID  EnableBusSupport=off  mask(LABCAR Outport){ModelName='Batterymodel_HiL', OutportID=9}
      mask help: This block defines an output of a Simulink model to another module of a LABCAR project
      settings: CopyFcn=set_param( gcb, 'UserData', '####');  OpenFcn=LCOpenFcnCallback
      mask Help:
      | Put this block onto any  hierarchy of the model and connect it to the model.
      | Rename it to any suitable name.
      | Then the corresponding signal is available in the Connection Manager for the wiring to any other module..
  Volt_10 : S-Function  FunctionName=LCOutport  Parameters=ModelName, OutportID  EnableBusSupport=off  mask(LABCAR Outport){ModelName='Batterymodel_HiL', OutportID=10}
      mask help: This block defines an output of a Simulink model to another module of a LABCAR project
      settings: CopyFcn=set_param( gcb, 'UserData', '####');  OpenFcn=LCOpenFcnCallback
      mask Help:
      | Put this block onto any  hierarchy of the model and connect it to the model.
      | Rename it to any suitable name.
      | Then the corresponding signal is available in the Connection Manager for the wiring to any other module..
  Volt_11 : S-Function  FunctionName=LCOutport  Parameters=ModelName, OutportID  EnableBusSupport=off  mask(LABCAR Outport){ModelName='Batterymodel_HiL', OutportID=11}
      mask help: This block defines an output of a Simulink model to another module of a LABCAR project
      settings: CopyFcn=set_param( gcb, 'UserData', '####');  OpenFcn=LCOpenFcnCallback
      mask Help:
      | Put this block onto any  hierarchy of the model and connect it to the model.
      | Rename it to any suitable name.
      | Then the corresponding signal is available in the Connection Manager for the wiring to any other module..
  Volt_12 : S-Function  FunctionName=LCOutport  Parameters=ModelName, OutportID  EnableBusSupport=off  mask(LABCAR Outport){ModelName='Batterymodel_HiL', OutportID=12}
      mask help: This block defines an output of a Simulink model to another module of a LABCAR project
      settings: CopyFcn=set_param( gcb, 'UserData', '####');  OpenFcn=LCOpenFcnCallback
      mask Help:
      | Put this block onto any  hierarchy of the model and connect it to the model.
      | Rename it to any suitable name.
      | Then the corresponding signal is available in the Connection Manager for the wiring to any other module..
  wires:
  Demux1/2 -> Volt_02/1
  Demux1/1 -> Volt_01/1
  Demux1/3 -> Volt_03/1
  Demux1/4 -> Volt_04/1
  Demux1/6 -> Volt_06/1
  Demux1/8 -> Volt_08/1
  Demux1/7 -> Volt_07/1
  Demux1/5 -> Volt_05/1
  Demux1/10 -> Volt_10/1
  Demux1/12 -> Volt_12/1
  Demux1/9 -> Volt_09/1
  Demux1/11 -> Volt_11/1
  cell_voltage [mV]/1 -> Demux1/1
